simulink model "sfcndemo_runtime"  (Simulink 6.0)
settings: Solver=FixedStepDiscrete  StartTime=0.0  StopTime=inf  RelTol=1e-3
PreLoadFcn:
  | gainVal=5;gainVal2=int8(5);
settings Model: CovMetricSettings=d  Creator=The MathWorks Inc.  LastModifiedBy=batserve  ExtModeAutoUpdateStatusClock=off  TunableVars=gainVal,gainVal2  TunableVarsStorageClass=Auto,Auto  TunableVarsTypeQualifier=,  ProdHWDeviceType=Specified
settings DataIOCC: SignalLoggingName=sigsOut
settings OptimizationCC: BlockReduction=off  BooleanDataType=off  InlineParams=on
settings DebuggingCC: CheckExecutionContextPreStartOutputMsg=on  CheckExecutionContextRuntimeOutputMsg=on  SolverPrmCheckMsg=none
settings HardwareCC: ProdBitPerShort=32  ProdBitPerInt=16  ProdHWDeviceType=Specified  TargetUnknown=on
settings RTWCC: RetainRTWFile=on

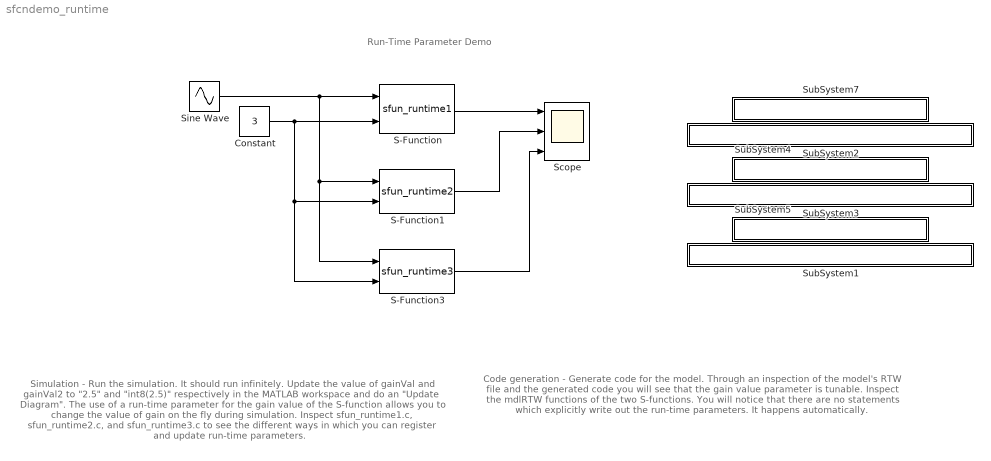
== system sfcndemo_runtime ==
  note: Run-Time Parameter Demo
  note: Simulation -
      | Run the simulation. It should run infinitely.
      | Update the value of gainVal and gainVal2 to "2.5" and
      | "int8(2.5)" respectively in the MATLAB workspace and do an
      | "Update Diagram". The use of a run-time parameter for the
      | gain value of the S-function allows you to change the value of
      | gain on the fly during simulation.
      |
      | Inspect sfun_runtime1.c, sfun_runtime2.c, and sfun_runtime3.c
      | to see the different ways in which you can register and update
      | run-time parameters.
  note: Code generation -
      | Generate code for the model. Through an inspection of the
      | model's RTW file and the generated code you will see that the
      | gain value parameter is tunable.
      |
      | Inspect the mdlRTW functions of the two S-functions. You will
      | notice that there are no statements which explicitly write out the
      | run-time parameters. It happens automatically.
  Constant : Constant  Value=3
  S-Function : S-Function  FunctionName=sfun_runtime1  Parameters='++',gainVal,'SumTimesGain'
  S-Function1 : S-Function  FunctionName=sfun_runtime2  Parameters='++',gainVal,'SumTimesGain'
  S-Function3 : S-Function  FunctionName=sfun_runtime3  Parameters='++',gainVal2,'SumTimesGain'
  Scope : Scope  NumInputPorts=3
      settings: TimeRange=4  YMin=5~5~5  YMax=20~20~20
  Sine Wave : Sin  SampleTime=0.1
  SubSystem1 : Subsystem  PropExecContextAcrossSSBoundary=on  mask{filename=sfun_runtime3.tlc}
      mask prompts: filename "file name"
      mask init:
      | x=sfundemo_maskdisp;
      settings: AttributesFormatString=\n\n\n\n\n\n\n\n\n\n  OpenFcn=sfundemo_openfcn
      mask Display: disp(x)
  SubSystem2 : Subsystem  PropExecContextAcrossSSBoundary=on  mask{filename=sfun_runtime1.tlc}
      mask prompts: filename "file name"
      mask init:
      | x=sfundemo_maskdisp;
      settings: AttributesFormatString=\n\n\n\n\n\n\n\n\n\n  OpenFcn=sfundemo_openfcn
      mask Display: disp(x)
  SubSystem3 : Subsystem  PropExecContextAcrossSSBoundary=on  mask{filename=sfun_runtime2.tlc}
      mask prompts: filename "file name"
      mask init:
      | x=sfundemo_maskdisp;
      settings: AttributesFormatString=\n\n\n\n\n\n\n\n\n\n  OpenFcn=sfundemo_openfcn
      mask Display: disp(x)
  SubSystem4 : Subsystem  PropExecContextAcrossSSBoundary=on  mask{filename=sfun_runtime2.c}
      mask prompts: filename "file name"
      mask init:
      | x=sfundemo_maskdisp;
      settings: AttributesFormatString=\n\n\n\n\n\n\n\n\n\n  OpenFcn=sfundemo_openfcn
      mask Display: disp(x)
  SubSystem5 : Subsystem  PropExecContextAcrossSSBoundary=on  mask{filename=sfun_runtime3.c}
      mask prompts: filename "file name"
      mask init:
      | x=sfundemo_maskdisp;
      settings: AttributesFormatString=\n\n\n\n\n\n\n\n\n\n  OpenFcn=sfundemo_openfcn
      mask Display: disp(x)
  SubSystem7 : Subsystem  PropExecContextAcrossSSBoundary=on  mask{filename=sfun_runtime1.c}
      mask prompts: filename "file name"
      mask init:
      | x=sfundemo_maskdisp;
      settings: AttributesFormatString=\n\n\n\n\n\n\n\n\n\n  OpenFcn=sfundemo_openfcn
      mask Display: disp(x)
  wires:
  Sine Wave/1 -> S-Function/1, S-Function1/1, S-Function3/1
  Constant/1 -> S-Function/2, S-Function1/2, S-Function3/2
  S-Function/1 -> Scope/1
  S-Function1/1 -> Scope/2
  S-Function3/1 -> Scope/3

== system sfcndemo_runtime/SubSystem1 ==

== system sfcndemo_runtime/SubSystem2 ==

== system sfcndemo_runtime/SubSystem3 ==

== system sfcndemo_runtime/SubSystem4 ==

== system sfcndemo_runtime/SubSystem5 ==

== system sfcndemo_runtime/SubSystem7 ==
